simulink library "rwa_zero_torque_power_lib"  (R2018b)
settings: Solver=VariableStepAuto  StartTime=0.0  StopTime=10.0  RelTol=1e-3
undefined symbols (not defined in the file): simParams
libraries: simulink x1
settings Model: Creator=Taylor  LastModifiedBy=Taylor

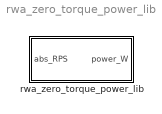
== system rwa_zero_torque_power_lib ==
  rwa_zero_torque_power_lib : Subsystem

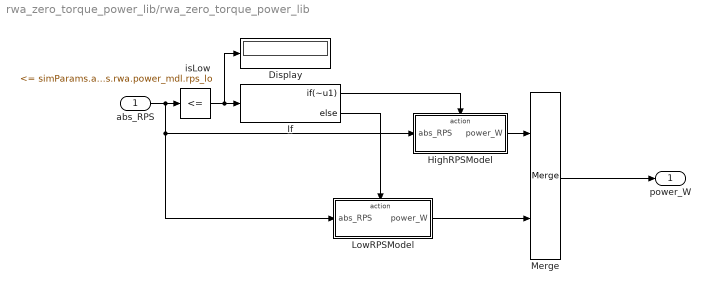
== system rwa_zero_torque_power_lib/rwa_zero_torque_power_lib ==
  abs_RPS : Inport
  Display : Display
  HighRPSModel : Subsystem  TreatAsAtomicUnit=on
  If : If  IfExpression=~u1
  LowRPSModel : Subsystem  TreatAsAtomicUnit=on
  Merge : Merge
  isLow : simulink/Logic and Bit Operations/Compare To Constant  relop=<=  const=simParams.actuators.rwa.power_mdl.rps_lo  OutDataTypeStr=boolean
  power_W : Outport
  wires:
  isLow/1 -> If/1, Display/1
  abs_RPS/1 -> LowRPSModel/1(abs_RPS), HighRPSModel/1(abs_RPS), isLow/1
  If/1 -> HighRPSModel/Action
  If/2 -> LowRPSModel/Action
  HighRPSModel/1(power_W) -> Merge/1
  LowRPSModel/1(power_W) -> Merge/2
  Merge/1 -> power_W/1

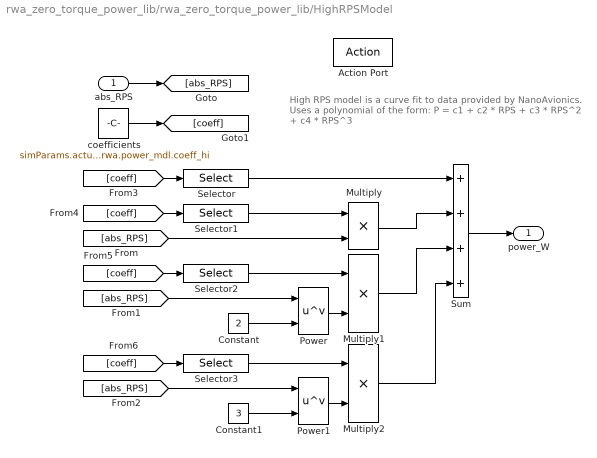
== system rwa_zero_torque_power_lib/rwa_zero_torque_power_lib/HighRPSModel ==
  note: High RPS model is a curve fit to data
      | provided by NanoAvionics. Uses a polynomial
      | of the form:
      | P = c1 + c2 * RPS + c3 * RPS^2 + c4 * RPS^3
  abs_RPS : Inport
  Action Port : ActionPort
  Constant : Constant  Value=2
  Constant1 : Constant  Value=3
  Multiply : Product
  Multiply1 : Product
  Multiply2 : Product
  Power : Math  Operator=pow  OutputSignalType=real  SaturateOnIntegerOverflow=on
  Power1 : Math  Operator=pow  OutputSignalType=real  SaturateOnIntegerOverflow=on
  Selector : Selector  InputPortWidth=4  IndexOptions=Index vector (dialog)  Indices=1  OutputSizes=1
  Selector1 : Selector  InputPortWidth=4  IndexOptions=Index vector (dialog)  Indices=2  OutputSizes=1
  Selector2 : Selector  InputPortWidth=4  IndexOptions=Index vector (dialog)  Indices=3  OutputSizes=1
  Selector3 : Selector  InputPortWidth=4  IndexOptions=Index vector (dialog)  Indices=4  OutputSizes=1
  Sum : Sum  Inputs=++++
  coefficients : Constant  Value=simParams.actuators.rwa.power_mdl.coeff_hi
  power_W : Outport
  wires:
  Selector/1 -> Sum/1
  abs_RPS/1 -> [abs_RPS]
  Selector1/1 -> Multiply/1
  [abs_RPS] -> Multiply/2
  [abs_RPS] -> Power/1
  Constant/1 -> Power/2
  Selector2/1 -> Multiply1/1
  Power/1 -> Multiply1/2
  Power1/1 -> Multiply2/2
  Selector3/1 -> Multiply2/1
  Constant1/1 -> Power1/2
  [abs_RPS] -> Power1/1
  Multiply/1 -> Sum/2
  Multiply1/1 -> Sum/3
  Multiply2/1 -> Sum/4
  Sum/1 -> power_W/1
  coefficients/1 -> [coeff]
  [coeff] -> Selector/1
  [coeff] -> Selector1/1
  [coeff] -> Selector2/1
  [coeff] -> Selector3/1

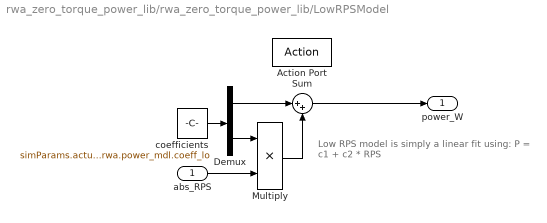
== system rwa_zero_torque_power_lib/rwa_zero_torque_power_lib/LowRPSModel ==
  note: Low RPS model is simply a linear
      | fit using:
      | P = c1 + c2 * RPS
  abs_RPS : Inport
  Action Port : ActionPort
  Demux : Demux  Outputs=2
  Multiply : Product
  Sum : Sum  Inputs=|++
  coefficients : Constant  Value=simParams.actuators.rwa.power_mdl.coeff_lo
  power_W : Outport
  wires:
  abs_RPS/1 -> Multiply/2
  Sum/1 -> power_W/1
  coefficients/1 -> Demux/1
  Demux/1 -> Sum/1
  Demux/2 -> Multiply/1
  Multiply/1 -> Sum/2
